simulink model "LQfullcar"  (R2022b)
settings: Solver=ode23tb  StartTime=0.0  StopTime=tsim  RelTol=1e-1
values from neighbouring files (symbols this model uses):
  A = [alpha*u zeros(1,4) ... (first row only)    [LQR.m]    (also in empc.m; lqrfullcar.m = [zeros(4,4) A12 zeros(4,4) -eye(4); A21 zeros(3,3) zeros(3,4; mpcfullcar.m = [zeros(4,4) A12 zeros(4,4) -eye(4); A21 zeros(3,3) zeros(3,4)
  alpha = -2*pi*n00    (= -11.88)    [LQR.m]    (also in empc.m; lqrfullcar.m; mpcfullcar.m)
  B = [0 ... (first row only)    [LQR.m]    (also in empc.m; lqrfullcar.m = [zeros(4,4); B21; zeros(4,4);B41]; mpcfullcar.m = [zeros(4,4); B21; zeros(4,4);B41])
  beta = 2*pi*n0*sqrt(Gn0)    [LQR.m]    (also in empc.m; lqrfullcar.m; mpcfullcar.m)
  C = [0 -ks/ms 0  ks/ms 0 ]    [LQR.m]    (also in empc.m; lqrfullcar.m = [C11 zeros(4,11)]; mpcfullcar.m = [C11 zeros(4,11)])
  Cy = [0 0 1 0 -1]    [LQR.m]    (also in empc.m; lqrfullcar.m = [C12 zeros(8,11)]; mpcfullcar.m = [C12 zeros(8,11)])
  D = zeros(4,4)    [lqrfullcar.m]    (also in mpcfullcar.m)
  Dyu = 0    [LQR.m]    (also in empc.m; lqrfullcar.m = [zeros(4,4);D11]; mpcfullcar.m = [zeros(4,4);D11])
  Dyw = zeros(8,4)    [lqrfullcar.m]    (also in mpcfullcar.m)
  E = [beta*sqrt(u) ... (first row only)    [LQR.m]    (also in empc.m; lqrfullcar.m = [zeros(4,4); zeros(3,4);-eye(4);zeros(4,4)]; mpcfullcar.m = [zeros(4,4); zeros(3,4);-eye(4);zeros(4,4)])
  F = F+trace(phi*Xtilde)    [empc.m]    (also in lqrfullcar.m = zeros(4,4); mpcfullcar.m)
  Kcl = [-0.15638609904 0.402772303704 0.258799770754 1.00139223609 -0.21001614058 -0.364861682479 0.0838087208096 -0.132385484064 -0.331025915395 -0.160574853071 -0.160142399635 0.494573338001 ... (60 elements, 4x15)]    [Kfull.mat]    (also in lqrfullcar.m = double(Y)/double(P))
  ktf = 228000    [LQR.m]    (also in empc.m; lqrfullcar.m; mpcfullcar.m)
  ktr = 228000    [LQR.m]    (also in empc.m; lqrfullcar.m; mpcfullcar.m)
  Kv = 48    [lqrfullcar.m]    (also in mpcfullcar.m)
  La = 0.003    [LQR.m]    (also in empc.m; lqrfullcar.m; mpcfullcar.m)
  Ra = 6    [LQR.m]    (also in empc.m; lqrfullcar.m; mpcfullcar.m)
  set_p = [ms;muf;mur;Ip;Ir;kf;kr;t_f;tr;ktf;ktr;bf;br;a;b]    [lqrfullcar.m]    (also in mpcfullcar.m)
libraries: spsMeanLib x12, dspstat3 x2
settings Model: Creator=simon  LastModifiedBy=HP
settings SolverCC: AlgebraicLoopSolver=TrustRegion
settings DataIOCC: ReturnWorkspaceOutputs=off
settings DebuggingCC: UnconnectedInputMsg=warning  UnconnectedOutputMsg=warning  UnconnectedLineMsg=warning  SFMachineParentedDataDiag=warning  ArithmeticOperatorsInVariantConditions=warning
settings ModelReferenceCC: EnableRefExpFcnMdlSchedulingChecks=on
settings SFSimCC: SimUseLocalCustomCode=off  CustomCodeUndefinedFunction=UseInterfaceOnly
settings RTWCC: RTWUseLocalCustomCode=off  DLArmComputeVersion=19.05

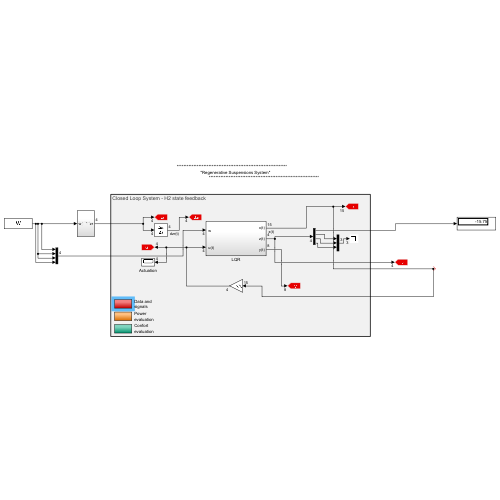
[thumbnail: Simulink's stored preview of the top-level diagram]
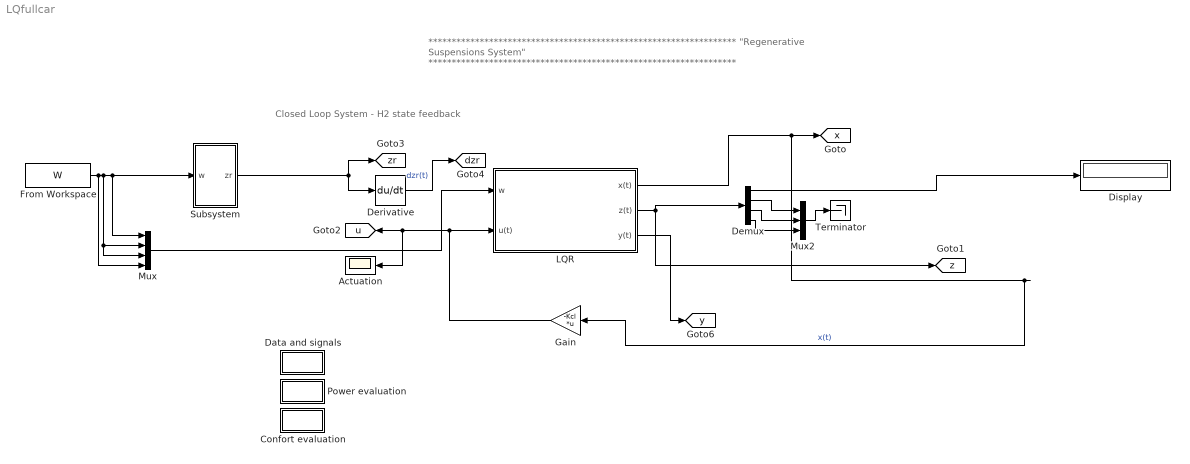
== system LQfullcar ==
  note: ******************************************************************
      | "Regenerative Suspensions System"
      | ******************************************************************
  note: Closed Loop System - H2 state feedback
  Actuation : Scope
  Confort evaluation : Subsystem
  Data and signals : Subsystem
  Demux : Demux
  Derivative : Derivative
  Display : Display
  From Workspace : FromWorkspace  VariableName=W
  Gain : Gain  Gain=-Kcl  Multiplication=Matrix(K*u)
  LQR : Subsystem
  Mux : Mux
  Mux2 : Mux  Inputs=3
  Power evaluation : Subsystem
  Subsystem : Subsystem
  Terminator : Terminator
  tag scope: dzr=global, u=global, x=global, y=global, z=global, zr=global
  wires:
  LQR/1(x(t)) -> Gain/1, [x]  "x(t)"
  Subsystem/1(zr) -> Derivative/1, [zr]
  Derivative/1 -> [dzr]  "dzr(t)"
  Gain/1 -> Actuation/1, [u], LQR/2(" u(t)")
  From Workspace/1 -> Mux/4, Mux/3, Mux/2, Mux/1, Subsystem/1(w)
  LQR/3(y(t)) -> [y]
  Mux/1 -> LQR/1(" w")
  LQR/2(z(t)) -> [z], Demux/1
  Demux/1 -> Display/1
  Demux/2 -> Mux2/1
  Demux/3 -> Mux2/2
  Demux/4 -> Mux2/3
  Mux2/1 -> Terminator/1

== system LQfullcar/Confort evaluation ==
  Demux : Demux  Outputs=[4 4]
  Display : Display
  RMS1 : dspstat3/RMS  run=on  directionMode=Each column  dimension=1  InputProcessing=Columns as channels (frame based)  reset_popup=None
  Terminator : Terminator
  Zero-Order Hold : ZeroOrderHold  SampleTime=0.001
  aw(t) : Scope
  tag scope: RI=global
  wires:
  [ztilde] -> Demux/1
  Zero-Order Hold/1 -> RMS1/1, aw(t)/1
  RMS1/1 -> [RI], Display/1  "RI"
  Demux/1 -> Zero-Order Hold/1  "aw(t)"
  Demux/2 -> Terminator/1

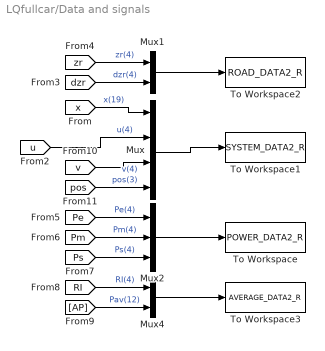
== system LQfullcar/Data and signals ==
  Mux : Mux
  Mux1 : Mux  Inputs=2
  Mux2 : Mux  Inputs=3
  Mux4 : Mux  Inputs=2
  To Workspace : ToWorkspace  VariableName=POWER_DATA2_R  SampleTime=-1
  To Workspace1 : ToWorkspace  VariableName=SYSTEM_DATA2_R  SampleTime=-1
  To Workspace2 : ToWorkspace  VariableName=ROAD_DATA2_R  SampleTime=-1
  To Workspace3 : ToWorkspace  VariableName=AVERAGE_DATA2_R  SampleTime=-1
  wires:
  [x] -> Mux/1  "x(19)"
  [zr] -> Mux1/1  "zr(4)"
  [dzr] -> Mux1/2  "dzr(4)"
  Mux1/1 -> To Workspace2/1
  Mux/1 -> To Workspace1/1
  Mux2/1 -> To Workspace/1
  [Pe] -> Mux2/1  "Pe(4)"
  [Pm] -> Mux2/2  "Pm(4)"
  [Ps] -> Mux2/3  "Ps(4)"
  Mux4/1 -> To Workspace3/1
  [RI] -> Mux4/1  "RI(4)"
  [AP] -> Mux4/2  "Pav(12)"
  [u] -> Mux/2  "u(4)"
  [v] -> Mux/3  "v(4)"
  [pos] -> Mux/4  "pos(3)"

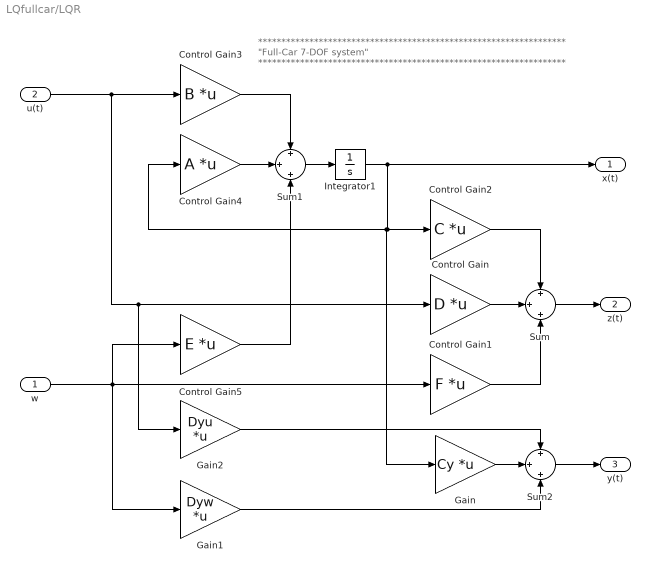
== system LQfullcar/LQR ==
  note: ******************************************************************
      |                            "Full-Car 7-DOF system"
      |
      | ******************************************************************
  " w" : Inport  PortDimensions=4
  " u(t)" : Inport  Port=2  PortDimensions=4
  Control Gain : Gain  Gain=D  Multiplication=Matrix(K*u)
  Control Gain1 : Gain  Gain=F  Multiplication=Matrix(K*u)
  Control Gain2 : Gain  Gain=C  Multiplication=Matrix(K*u)
  Control Gain3 : Gain  Gain=B  Multiplication=Matrix(K*u)
  Control Gain4 : Gain  Gain=A  Multiplication=Matrix(K*u)
  Control Gain5 : Gain  Gain=E  Multiplication=Matrix(K*u)
  Gain : Gain  Gain=Cy  Multiplication=Matrix(K*u)
  Gain1 : Gain  Gain=Dyw  Multiplication=Matrix(K*u)
  Gain2 : Gain  Gain=Dyu  Multiplication=Matrix(K*u)
  Integrator1 : Integrator
  Sum : Sum  Inputs=+|+|+
  Sum1 : Sum  Inputs=+|+|+
  Sum2 : Sum  Inputs=+|+|+
  x(t) : Outport  PortDimensions=15  VectorParamsAs1DForOutWhenUnconnected=off
  z(t) : Outport  Port=2  VectorParamsAs1DForOutWhenUnconnected=off
  y(t) : Outport  Port=3  VectorParamsAs1DForOutWhenUnconnected=off
  wires:
  Control Gain/1 -> Sum/2
  Control Gain2/1 -> Sum/1
  Control Gain1/1 -> Sum/3
  Control Gain3/1 -> Sum1/1
  Control Gain4/1 -> Sum1/2
  Sum1/1 -> Integrator1/1
  " u(t)"/1 -> Gain2/1, Control Gain/1, Control Gain3/1
  " w"/1 -> Gain1/1, Control Gain5/1, Control Gain1/1
  Control Gain5/1 -> Sum1/3
  Integrator1/1 -> x(t)/1, Gain/1, Control Gain4/1, Control Gain2/1
  Gain/1 -> Sum2/2
  Sum2/1 -> y(t)/1
  Gain1/1 -> Sum2/3
  Gain2/1 -> Sum2/1
  Sum/1 -> z(t)/1

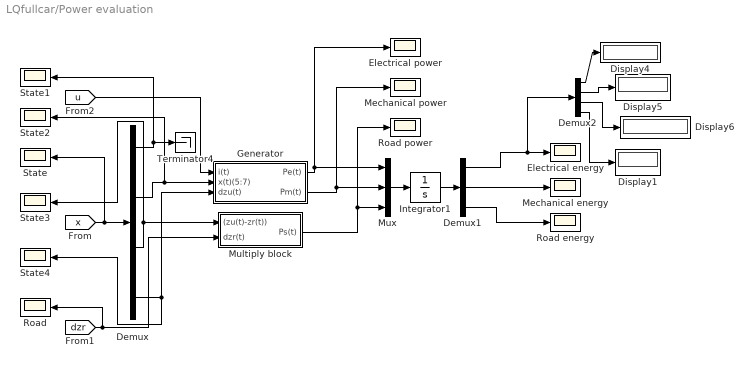
== system LQfullcar/Power evaluation ==
  Demux : Demux  Outputs=[4 3 4 4]
  Demux1 : Demux  Outputs=[4 4 4]
  Demux2 : Demux
  Display{1,4..6} (4 alike) : Display
  Electrical energy : Scope
  Electrical power : Scope
  Generator : Subsystem
  Integrator1 : Integrator
  Mechanical energy : Scope
  Mechanical power : Scope
  Multiply block : Subsystem
  Mux : Mux  Inputs=[4 4 4]
  Road : Scope
  Road energy : Scope
  Road power : Scope
  State{,1..4} (5 alike) : Scope
  Terminator4 : Terminator
  wires:
  Multiply block/1(Ps(t)) -> Mux/3, Road power/1
  [x] -> State/1, Demux/1
  Demux/3 -> Multiply block/1((zu(t)-zr(t))), State3/1
  [dzr] -> Multiply block/2(dzr(t)), Road/1
  Demux/2 -> Generator/2(x(t)(5:7)), State2/1
  Mux/1 -> Integrator1/1
  Demux/1 -> State1/1, Terminator4/1
  [u] -> Generator/1(i(t))
  Demux1/2 -> Mechanical energy/1
  Generator/2(Pm(t)) -> Mechanical power/1, Mux/2
  Generator/1(Pe(t)) -> Mux/1, Electrical power/1
  Demux/4 -> Generator/3(dzu(t)), State4/1
  Integrator1/1 -> Demux1/1
  Demux1/3 -> Road energy/1
  Demux2/4 -> Display1/1
  Demux2/3 -> Display6/1
  Demux2/1 -> Display4/1
  Demux1/1 -> Demux2/1, Electrical energy/1
  Demux2/2 -> Display5/1

== system LQfullcar/Subsystem ==
  note: alpha*u*zr
  note: zdotr
  note: zr
  w : Inport
  Gain : Gain  Gain=beta*sqrt(u)
  Gain1 : Gain  Gain=alpha*u
  Integrator : Integrator
  Mux : Mux
  Scope : Scope
  Sum : Sum  Inputs=|++
  zr : Outport
  wires:
  w/1 -> Gain/1
  Gain1/1 -> Sum/1
  Sum/1 -> Integrator/1
  Integrator/1 -> Mux/1, Mux/4, Scope/1, Mux/3, Mux/2, Gain1/1
  Gain/1 -> Sum/2
  Mux/1 -> zr/1

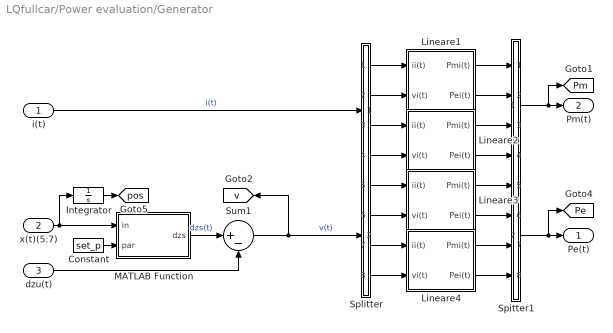
== system LQfullcar/Power evaluation/Generator ==
  i(t) : Inport
  x(t)(5:7) : Inport  Port=2
  dzu(t) : Inport  Port=3
  Constant : Constant  Value=set_p
  Integrator : Integrator
  Lineare1 : Subsystem
  Lineare2 : Subsystem
  Lineare3 : Subsystem
  Lineare4 : Subsystem
  MATLAB Function : MATLAB Function  TreatAsAtomicUnit=on
  Spitter1 : Subsystem
  Splitter : Subsystem
  Sum1 : Sum  Inputs=|+-
  Pe(t) : Outport  VectorParamsAs1DForOutWhenUnconnected=off
  Pm(t) : Outport  Port=2  VectorParamsAs1DForOutWhenUnconnected=off
  tag scope: Pe=global, Pm=global, pos=global, v=global
  wires:
  Lineare2/2(Pei(t)) -> Spitter1/4(In4)
  Lineare1/2(Pei(t)) -> Spitter1/2(In2)
  Lineare3/1(Pmi(t)) -> Spitter1/5(In5)
  x(t)(5:7)/1 -> MATLAB Function/1(in), Integrator/1
  Constant/1 -> MATLAB Function/2(par)
  Splitter/2(Out2) -> Lineare1/2(vi(t))
  Splitter/5(Out5) -> Lineare3/1(ii(t))
  Splitter/7(Out7) -> Lineare4/1(ii(t))
  Sum1/1 -> [v], Splitter/2(v(t))  "v(t)"
  Lineare2/1(Pmi(t)) -> Spitter1/3(In3)
  Spitter1/2(Pe(t)) -> [Pe], Pe(t)/1
  Splitter/3(Out3) -> Lineare2/1(ii(t))
  Integrator/1 -> [pos]
  Lineare4/1(Pmi(t)) -> Spitter1/7(In7)
  Splitter/4(Out4) -> Lineare2/2(vi(t))
  Splitter/8(Out8) -> Lineare4/2(vi(t))
  Splitter/6(Out6) -> Lineare3/2(vi(t))
  Lineare4/2(Pei(t)) -> Spitter1/8(In8)
  Lineare3/2(Pei(t)) -> Spitter1/6(In6)
  Spitter1/1(Pm(t)) -> Pm(t)/1, [Pm]
  MATLAB Function/1(dzs) -> Sum1/1  "dzs(t)"
  dzu(t)/1 -> Sum1/2
  i(t)/1 -> Splitter/1(i(t))  "i(t)"
  Lineare1/1(Pmi(t)) -> Spitter1/1(In1)
  Splitter/1(Out1) -> Lineare1/1(ii(t))

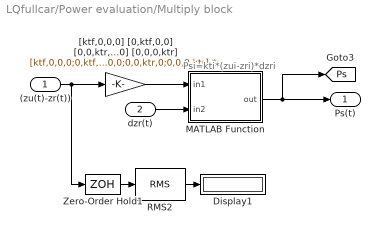
== system LQfullcar/Power evaluation/Multiply block ==
  note: Psi=kti*(zui-zri)*dzri
  (zu(t)-zr(t)) : Inport
  dzr(t) : Inport  Port=2
  Display1 : Display
      settings: Format=short_e
  MATLAB Function : MATLAB Function  TreatAsAtomicUnit=on
  RMS2 : dspstat3/RMS  run=on  directionMode=Each column  dimension=1  InputProcessing=Columns as channels (frame based)  reset_popup=None
  Zero-Order Hold1 : ZeroOrderHold  SampleTime=0.001
  "[ktf,0,0,0] [0,ktf,0,0] [0,0,ktr,0] [0,0,0,ktr]" : Gain  Gain=[ktf,0,0,0;0,ktf,0,0;0,0,ktr,0;0,0,0,ktr]  Multiplication=Matrix(K*u)
  Ps(t) : Outport  VectorParamsAs1DForOutWhenUnconnected=off
  tag scope: Ps=global
  wires:
  dzr(t)/1 -> MATLAB Function/2(in2)
  (zu(t)-zr(t))/1 -> Zero-Order Hold1/1, "[ktf,0,0,0] [0,ktf,0,0] [0,0,ktr,0] [0,0,0,ktr]"/1
  MATLAB Function/1(out) -> [Ps], Ps(t)/1
  "[ktf,0,0,0] [0,ktf,0,0] [0,0,ktr,0] [0,0,0,ktr]"/1 -> MATLAB Function/1(in1)
  Zero-Order Hold1/1 -> RMS2/1
  RMS2/1 -> Display1/1

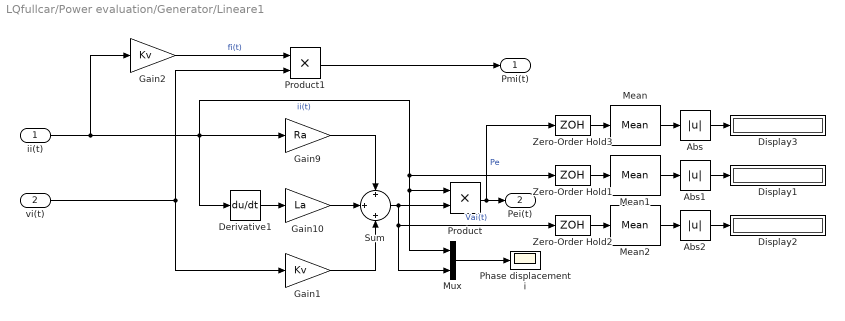
== system LQfullcar/Power evaluation/Generator/Lineare1 ==
  ii(t) : Inport
  vi(t) : Inport  Port=2
  Abs : Abs  SaturateOnIntegerOverflow=off
  Abs1 : Abs  SaturateOnIntegerOverflow=off
  Abs2 : Abs  SaturateOnIntegerOverflow=off
  Derivative1 : Derivative
  Display1 : Display
  Display2 : Display
  Display3 : Display
  Gain1 : Gain  Gain=Kv
  Gain10 : Gain  Gain=La
  Gain2 : Gain  Gain=Kv
  Gain9 : Gain  Gain=Ra
  Mean : spsMeanLib/Mean  Freq=60  Vinit=0  Ts=0
  Mean1 : spsMeanLib/Mean  Freq=60  Vinit=0  Ts=0
  Mean2 : spsMeanLib/Mean  Freq=60  Vinit=0  Ts=0
  Mux : Mux  Inputs=2
  Phase displacement i : Scope
  Product : Product  RndMeth=Zero
  Product1 : Product  RndMeth=Zero
  Sum : Sum  Inputs=+|+|+
  Zero-Order Hold1 : ZeroOrderHold  SampleTime=0.001
  Zero-Order Hold2 : ZeroOrderHold  SampleTime=0.001
  Zero-Order Hold3 : ZeroOrderHold  SampleTime=0.001
  Pmi(t) : Outport  VectorParamsAs1DForOutWhenUnconnected=off
  Pei(t) : Outport  Port=2  VectorParamsAs1DForOutWhenUnconnected=off
  wires:
  Derivative1/1 -> Gain10/1
  Gain9/1 -> Sum/1
  Gain10/1 -> Sum/2
  Gain1/1 -> Sum/3
  Product/1 -> Zero-Order Hold3/1, Pei(t)/1  "Pe"
  vi(t)/1 -> Gain1/1, Product1/2
  Mux/1 -> Phase displacement i/1
  Product1/1 -> Pmi(t)/1
  Gain2/1 -> Product1/1  "fi(t)"
  Sum/1 -> Product/2, Zero-Order Hold2/1, Mux/2  "Vai(t)"
  Zero-Order Hold1/1 -> Mean1/1
  ii(t)/1 -> Gain2/1, Gain9/1, Zero-Order Hold1/1, Mux/1, Product/1, Derivative1/1  "ii(t)"
  Zero-Order Hold2/1 -> Mean2/1
  Zero-Order Hold3/1 -> Mean/1
  Mean/1 -> Abs/1
  Abs/1 -> Display3/1
  Mean1/1 -> Abs1/1
  Abs1/1 -> Display1/1
  Mean2/1 -> Abs2/1
  Abs2/1 -> Display2/1

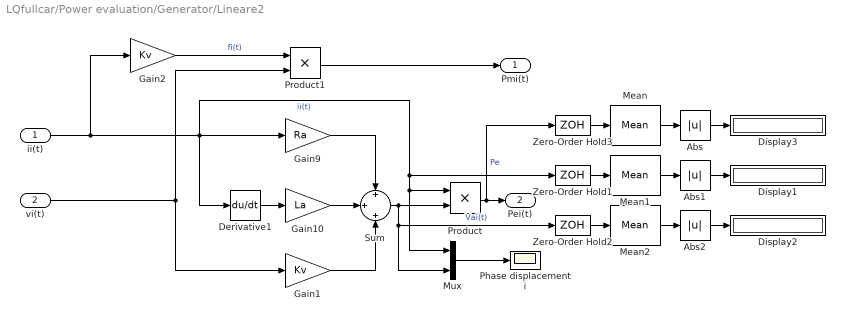
== system LQfullcar/Power evaluation/Generator/Lineare2 ==
  ii(t) : Inport
  vi(t) : Inport  Port=2
  Abs : Abs  SaturateOnIntegerOverflow=off
  Abs1 : Abs  SaturateOnIntegerOverflow=off
  Abs2 : Abs  SaturateOnIntegerOverflow=off
  Derivative1 : Derivative
  Display1 : Display
  Display2 : Display
  Display3 : Display
  Gain1 : Gain  Gain=Kv
  Gain10 : Gain  Gain=La
  Gain2 : Gain  Gain=Kv
  Gain9 : Gain  Gain=Ra
  Mean : spsMeanLib/Mean  Freq=60  Vinit=0  Ts=0
  Mean1 : spsMeanLib/Mean  Freq=60  Vinit=0  Ts=0
  Mean2 : spsMeanLib/Mean  Freq=60  Vinit=0  Ts=0
  Mux : Mux  Inputs=2
  Phase displacement i : Scope
  Product : Product  RndMeth=Zero
  Product1 : Product  RndMeth=Zero
  Sum : Sum  Inputs=+|+|+
  Zero-Order Hold1 : ZeroOrderHold  SampleTime=0.001
  Zero-Order Hold2 : ZeroOrderHold  SampleTime=0.001
  Zero-Order Hold3 : ZeroOrderHold  SampleTime=0.001
  Pmi(t) : Outport  VectorParamsAs1DForOutWhenUnconnected=off
  Pei(t) : Outport  Port=2  VectorParamsAs1DForOutWhenUnconnected=off
  wires:
  Derivative1/1 -> Gain10/1
  Gain9/1 -> Sum/1
  Gain10/1 -> Sum/2
  Gain1/1 -> Sum/3
  Product/1 -> Zero-Order Hold3/1, Pei(t)/1  "Pe"
  vi(t)/1 -> Gain1/1, Product1/2
  Mux/1 -> Phase displacement i/1
  Product1/1 -> Pmi(t)/1
  Gain2/1 -> Product1/1  "fi(t)"
  Sum/1 -> Product/2, Zero-Order Hold2/1, Mux/2  "Vai(t)"
  Zero-Order Hold1/1 -> Mean1/1
  ii(t)/1 -> Gain2/1, Gain9/1, Zero-Order Hold1/1, Mux/1, Product/1, Derivative1/1  "ii(t)"
  Zero-Order Hold2/1 -> Mean2/1
  Zero-Order Hold3/1 -> Mean/1
  Mean/1 -> Abs/1
  Abs/1 -> Display3/1
  Mean1/1 -> Abs1/1
  Abs1/1 -> Display1/1
  Mean2/1 -> Abs2/1
  Abs2/1 -> Display2/1

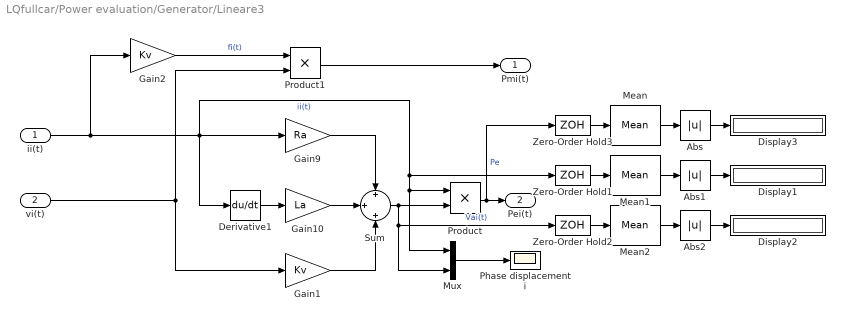
== system LQfullcar/Power evaluation/Generator/Lineare3 ==
  ii(t) : Inport
  vi(t) : Inport  Port=2
  Abs : Abs  SaturateOnIntegerOverflow=off
  Abs1 : Abs  SaturateOnIntegerOverflow=off
  Abs2 : Abs  SaturateOnIntegerOverflow=off
  Derivative1 : Derivative
  Display1 : Display
  Display2 : Display
  Display3 : Display
  Gain1 : Gain  Gain=Kv
  Gain10 : Gain  Gain=La
  Gain2 : Gain  Gain=Kv
  Gain9 : Gain  Gain=Ra
  Mean : spsMeanLib/Mean  Freq=60  Vinit=0  Ts=0
  Mean1 : spsMeanLib/Mean  Freq=60  Vinit=0  Ts=0
  Mean2 : spsMeanLib/Mean  Freq=60  Vinit=0  Ts=0
  Mux : Mux  Inputs=2
  Phase displacement i : Scope
  Product : Product  RndMeth=Zero
  Product1 : Product  RndMeth=Zero
  Sum : Sum  Inputs=+|+|+
  Zero-Order Hold1 : ZeroOrderHold  SampleTime=0.001
  Zero-Order Hold2 : ZeroOrderHold  SampleTime=0.001
  Zero-Order Hold3 : ZeroOrderHold  SampleTime=0.001
  Pmi(t) : Outport  VectorParamsAs1DForOutWhenUnconnected=off
  Pei(t) : Outport  Port=2  VectorParamsAs1DForOutWhenUnconnected=off
  wires:
  Derivative1/1 -> Gain10/1
  Gain9/1 -> Sum/1
  Gain10/1 -> Sum/2
  Gain1/1 -> Sum/3
  Product/1 -> Zero-Order Hold3/1, Pei(t)/1  "Pe"
  vi(t)/1 -> Gain1/1, Product1/2
  Mux/1 -> Phase displacement i/1
  Product1/1 -> Pmi(t)/1
  Gain2/1 -> Product1/1  "fi(t)"
  Sum/1 -> Product/2, Zero-Order Hold2/1, Mux/2  "Vai(t)"
  Zero-Order Hold1/1 -> Mean1/1
  ii(t)/1 -> Gain2/1, Gain9/1, Zero-Order Hold1/1, Mux/1, Product/1, Derivative1/1  "ii(t)"
  Zero-Order Hold2/1 -> Mean2/1
  Zero-Order Hold3/1 -> Mean/1
  Mean/1 -> Abs/1
  Abs/1 -> Display3/1
  Mean1/1 -> Abs1/1
  Mean2/1 -> Abs2/1
  Abs2/1 -> Display2/1
  Abs1/1 -> Display1/1

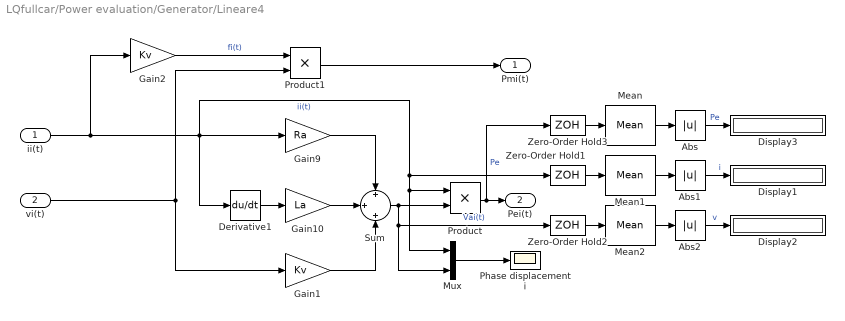
== system LQfullcar/Power evaluation/Generator/Lineare4 ==
  ii(t) : Inport
  vi(t) : Inport  Port=2
  Abs : Abs  SaturateOnIntegerOverflow=off
  Abs1 : Abs  SaturateOnIntegerOverflow=off
  Abs2 : Abs  SaturateOnIntegerOverflow=off
  Derivative1 : Derivative
  Display1 : Display
  Display2 : Display
  Display3 : Display
  Gain1 : Gain  Gain=Kv
  Gain10 : Gain  Gain=La
  Gain2 : Gain  Gain=Kv
  Gain9 : Gain  Gain=Ra
  Mean : spsMeanLib/Mean  Freq=60  Vinit=0  Ts=0
  Mean1 : spsMeanLib/Mean  Freq=60  Vinit=0  Ts=0
  Mean2 : spsMeanLib/Mean  Freq=60  Vinit=0  Ts=0
  Mux : Mux  Inputs=2
  Phase displacement i : Scope
  Product : Product  RndMeth=Zero
  Product1 : Product  RndMeth=Zero
  Sum : Sum  Inputs=+|+|+
  Zero-Order Hold1 : ZeroOrderHold  SampleTime=0.001
  Zero-Order Hold2 : ZeroOrderHold  SampleTime=0.001
  Zero-Order Hold3 : ZeroOrderHold  SampleTime=0.001
  Pmi(t) : Outport  VectorParamsAs1DForOutWhenUnconnected=off
  Pei(t) : Outport  Port=2  VectorParamsAs1DForOutWhenUnconnected=off
  wires:
  Derivative1/1 -> Gain10/1
  Gain9/1 -> Sum/1
  Gain10/1 -> Sum/2
  Gain1/1 -> Sum/3
  Product/1 -> Zero-Order Hold3/1, Pei(t)/1  "Pe"
  vi(t)/1 -> Gain1/1, Product1/2
  Mux/1 -> Phase displacement i/1
  Product1/1 -> Pmi(t)/1
  Gain2/1 -> Product1/1  "fi(t)"
  Sum/1 -> Product/2, Zero-Order Hold2/1, Mux/2  "Vai(t)"
  Zero-Order Hold1/1 -> Mean1/1
  ii(t)/1 -> Gain2/1, Gain9/1, Zero-Order Hold1/1, Mux/1, Product/1, Derivative1/1  "ii(t)"
  Zero-Order Hold2/1 -> Mean2/1
  Zero-Order Hold3/1 -> Mean/1
  Mean/1 -> Abs/1
  Abs/1 -> Display3/1  "Pe"
  Mean1/1 -> Abs1/1
  Abs1/1 -> Display1/1  "i"
  Abs2/1 -> Display2/1  "v"
  Mean2/1 -> Abs2/1

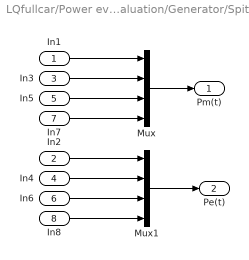
== system LQfullcar/Power evaluation/Generator/Spitter1 ==
  In1 : Inport
  In2 : Inport  Port=2
  In3 : Inport  Port=3
  In4 : Inport  Port=4
  In5 : Inport  Port=5
  In6 : Inport  Port=6
  In7 : Inport  Port=7
  In8 : Inport  Port=8
  Mux : Mux
  Mux1 : Mux
  Pm(t) : Outport  VectorParamsAs1DForOutWhenUnconnected=off
  Pe(t) : Outport  Port=2  VectorParamsAs1DForOutWhenUnconnected=off
  wires:
  In8/1 -> Mux1/4
  In2/1 -> Mux1/1
  Mux/1 -> Pm(t)/1
  In7/1 -> Mux/4
  In3/1 -> Mux/2
  In5/1 -> Mux/3
  Mux1/1 -> Pe(t)/1
  In1/1 -> Mux/1
  In6/1 -> Mux1/3
  In4/1 -> Mux1/2

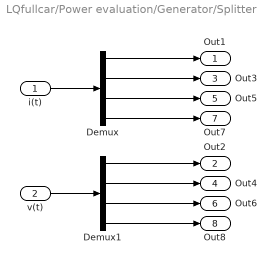
== system LQfullcar/Power evaluation/Generator/Splitter ==
  i(t) : Inport
  v(t) : Inport  Port=2
  Demux : Demux
  Demux1 : Demux
  Out1 : Outport  VectorParamsAs1DForOutWhenUnconnected=off
  Out2 : Outport  Port=2  VectorParamsAs1DForOutWhenUnconnected=off
  Out3 : Outport  Port=3  VectorParamsAs1DForOutWhenUnconnected=off
  Out4 : Outport  Port=4  VectorParamsAs1DForOutWhenUnconnected=off
  Out5 : Outport  Port=5  VectorParamsAs1DForOutWhenUnconnected=off
  Out6 : Outport  Port=6  VectorParamsAs1DForOutWhenUnconnected=off
  Out7 : Outport  Port=7  VectorParamsAs1DForOutWhenUnconnected=off
  Out8 : Outport  Port=8  VectorParamsAs1DForOutWhenUnconnected=off
  wires:
  i(t)/1 -> Demux/1
  Demux1/3 -> Out6/1
  Demux1/4 -> Out8/1
  Demux/1 -> Out1/1
  Demux1/2 -> Out4/1
  Demux1/1 -> Out2/1
  v(t)/1 -> Demux1/1
  Demux/2 -> Out3/1
  Demux/4 -> Out7/1
  Demux/3 -> Out5/1

== matlab function LQfullcar/Power evaluation/Multiply block/MATLAB Function ==
  data: in1 input; out output; in2 input
function out=fcn(in1,in2)

out1=in1(1)*in2(1);
out2=in1(2)*in2(2);
out3=in1(3)*in2(3);
out4=in1(4)*in2(4);

out=[out1;out2;out3;out4];

== matlab function LQfullcar/Power evaluation/Generator/MATLAB Function ==
  data: in input; dzs output; par input
function dzs=fcn(in,par)

dzs1=par(8)*in(1)+par(14)*in(2)+in(3);
dzs2=-par(8)*in(1)+par(14)*in(2)+in(3);
dzs3=par(9)*in(1)-par(15)*in(2)+in(3);
dzs4=-par(9)*in(1)-par(15)*in(2)+in(3);

dzs=[dzs1;dzs2;dzs3;dzs4];
